simulink model "b07502056_HW5_matlab"  (R2022a)
settings: Solver=VariableStepAuto  StartTime=0.0  StopTime=8  RelTol=1e-3
model workspace (MAT data in the model file):
  Engine_Breakpoint = Simulink.Parameter
  Engine_Breakpoint.Value = [1000 1500 2000 2500 3000 3500 4000 4500 5000 5500 6000 6500 7000 7500 8000 8500 9000]
  Engine_Breakpoint.DataType = 'auto'
  Engine_Breakpoint.Complexity = 'real'
  Engine_Breakpoint.Dimensions = [1 17]
  Engine_Torque = Simulink.Parameter
  Engine_Torque.Value = [850 850 850 850 850 850 850 830 820 770 700 650 600 560 525 490 470]
  Engine_Torque.DataType = 'auto'
  Engine_Torque.Complexity = 'real'
  Engine_Torque.Dimensions = [1 17]
  Final_Drive = 2.5
  Gear_Number = Simulink.Parameter
  Gear_Number.Value = [0 1 2]
  Gear_Number.DataType = 'auto'
  Gear_Number.Complexity = 'real'
  Gear_Number.Dimensions = [1 3]
  Gear_Ratio = Simulink.Parameter
  Gear_Ratio.Value = [-3.297 15.5 8.05]
  Gear_Ratio.DataType = 'auto'
  Gear_Ratio.Complexity = 'real'
  Gear_Ratio.Dimensions = [1 3]
  Pedal_Depth = 1
  Tyre = Simulink.Parameter
  Tyre.Value = [275 0.4 482.6]
  Tyre.DataType = 'auto'
  Tyre.Complexity = 'real'
  Tyre.Dimensions = [1 3]
libraries: vehdynlibviscommon x1, autolibshared x1
settings Model: PacingRate=0.800000  Creator=will  LastModifiedBy=will

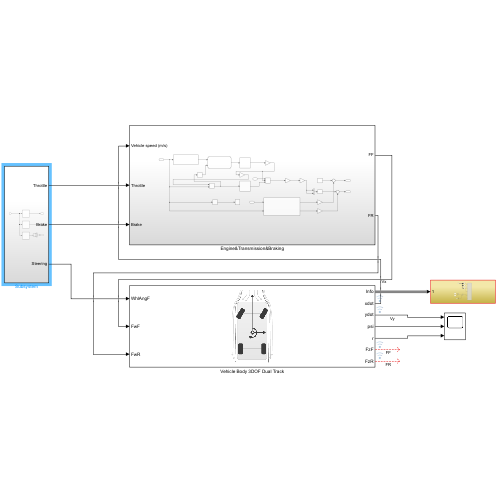
[thumbnail: Simulink's stored preview of the top-level diagram]
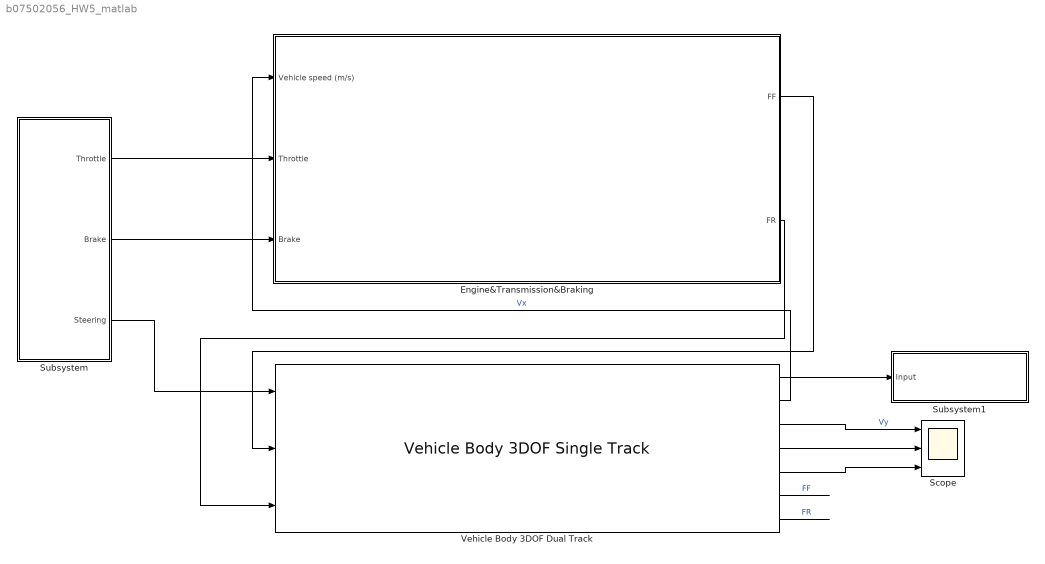
== system b07502056_HW5_matlab ==
  Engine&Transmission&Braking : Subsystem
  Scope : Scope  NumInputPorts=3
  Subsystem : Subsystem
  Subsystem1 : Subsystem
  Vehicle Body 3DOF Dual Track : autolibshared/Vehicle Body 3DOF Single Track  trackMode=Dual  inputMode=External longitudinal forces  frontSteerMode=on  rearSteerMode=off  windMode=off  muMode=off  extFMode=off  extMMode=off  htchFMode=off  htchMMode=off  extXo=off  extpsio=off  extxdoto=off  extro=off  extYo=off  extTamb=off  extydoto=off  aMode=2  NF=2  NR=2  m=2295  a=1.45  b=1.45  h=0.3  dh=1  hh=0.2  X_o=0  xdot_o=0  CalphaMode=off  sigmaMode=on  d=0  hl=0  w=[1.4,1.4]  Cy_f=12e3  Cy_r=11e3  sigma_f=.1  sigma_r=.1  alpha_f_brk=[-.1 .1]  Cy_f_data=[-9e3 9e3]  alpha_r_brk=[-.1 .1]  Cy_r_data=[-9e3 9e3]  Y_o=0  ydot_o=0  Izz=4000  psi_o=0  r_o=0  Af=2.33  Cd=.22  Cl=.1  Cpm=.1  beta_w=[0 0.01:0.01:0.3]  Cs=[0:0.03:0.9]  Cym=[0 1e-6:0.01:0.3]  Pabs=101325  Tair=273  g=9.81  mu=1  xdot_tol=.01  Fznom=5000  Fxtire_sat=7e4  Fytire_sat=7e4  longOff=0  latOff=0  vertOff=0  wrapAng=off
      settings: SourceProductBaseCode=PW,DR,MT,VE
  wires:
  Vehicle Body 3DOF Dual Track/2 -> Engine&Transmission&Braking/1(Vehicle speed (m/s))  "Vx"
  Subsystem/1(Throttle) -> Engine&Transmission&Braking/2(Throttle)
  Engine&Transmission&Braking/2(FR) -> Vehicle Body 3DOF Dual Track/3
  Engine&Transmission&Braking/1(FF) -> Vehicle Body 3DOF Dual Track/2
  Subsystem/2(Brake) -> Engine&Transmission&Braking/3(Brake)
  Subsystem/3(Steering) -> Vehicle Body 3DOF Dual Track/1
  Vehicle Body 3DOF Dual Track/3 -> Scope/1  "Vy"
  Vehicle Body 3DOF Dual Track/4 -> Scope/2
  Vehicle Body 3DOF Dual Track/5 -> Scope/3
  Vehicle Body 3DOF Dual Track/1 -> Subsystem1/1(Input)
  Vehicle Body 3DOF Dual Track/6 -> ?  "FF"
  Vehicle Body 3DOF Dual Track/7 -> ?  "FR"

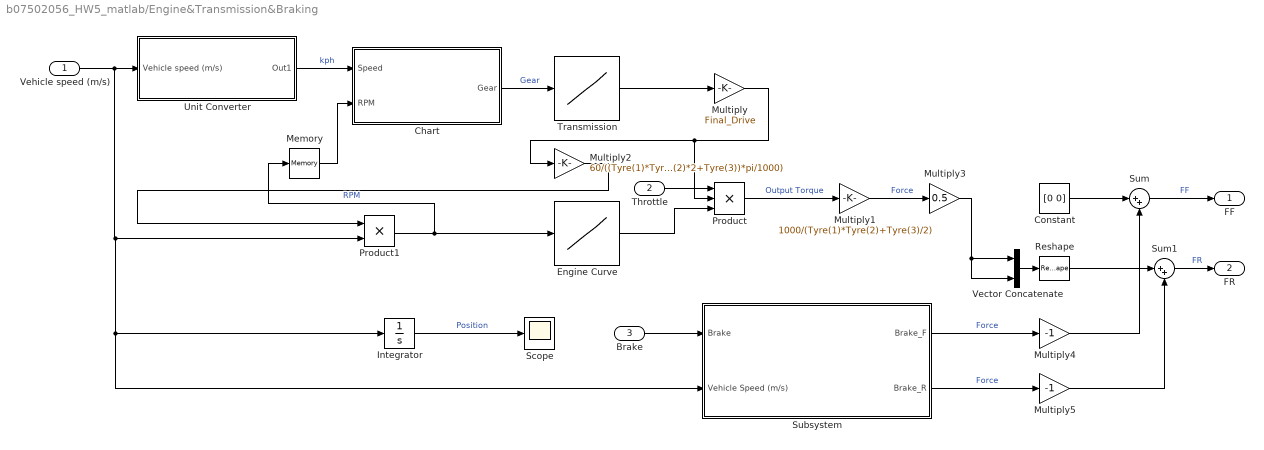
== system b07502056_HW5_matlab/Engine&Transmission&Braking ==
  Vehicle speed (m/s) : Inport
  Throttle : Inport  Port=2
  Brake : Inport  Port=3
  Chart : Stateflow chart  TreatAsAtomicUnit=on
  Constant : Constant  Value=[0 0]
  Engine Curve : Lookup_n-D  NumberOfTableDimensions=1  BreakpointsForDimension1=Engine_Breakpoint  Table=Engine_Torque  InternalRulePriority=Speed  RndMeth=Simplest
  Integrator : Integrator
  Memory : Memory
  Multiply : Gain  Gain=Final_Drive
  Multiply1 : Gain  Gain=1000/(Tyre(1)*Tyre(2)+Tyre(3)/2)
  Multiply2 : Gain  Gain=60/((Tyre(1)*Tyre(2)*2+Tyre(3))*pi/1000)
  Multiply3 : Gain  Gain=0.5
  Multiply4 : Gain  Gain=-1
  Multiply5 : Gain  Gain=-1
  Product : Product  Inputs=3
  Product1 : Product
  Reshape : Reshape
  Scope : Scope
  Subsystem : Subsystem
  Sum : Sum  Inputs=|++
  Sum1 : Sum  Inputs=|++
  Transmission : Lookup_n-D  NumberOfTableDimensions=1  BreakpointsForDimension1=Gear_Number  Table=Gear_Ratio  InternalRulePriority=Speed  RndMeth=Simplest
  Unit Converter : Subsystem
  Vector Concatenate : Concatenate
  FF : Outport
  FR : Outport  Port=2
  wires:
  Chart/1(Gear) -> Transmission/1  "Gear"
  Vehicle speed (m/s)/1 -> Subsystem/2(Vehicle Speed (m/s)), Integrator/1, Product1/2, Unit Converter/1(Vehicle speed (m/s))
  Unit Converter/1(Out1) -> Chart/1(Speed)  "kph"
  Engine Curve/1 -> Product/3
  Transmission/1 -> Multiply/1
  Throttle/1 -> Product/1
  Product/1 -> Multiply1/1  "Output Torque"
  Multiply/1 -> Product/2, Multiply2/1
  Multiply2/1 -> Product1/1
  Product1/1 -> Memory/1, Engine Curve/1  "RPM"
  Memory/1 -> Chart/2(RPM)
  Integrator/1 -> Scope/1  "Position"
  Multiply1/1 -> Multiply3/1  "Force"
  Vector Concatenate/1 -> Reshape/1
  Multiply3/1 -> Vector Concatenate/1, Vector Concatenate/2
  Brake/1 -> Subsystem/1(Brake)
  Sum1/1 -> FR/1  "FR"
  Reshape/1 -> Sum1/1
  Sum/1 -> FF/1  "FF"
  Constant/1 -> Sum/1
  Multiply4/1 -> Sum/2
  Multiply5/1 -> Sum1/2
  Subsystem/1(Brake_F) -> Multiply4/1  "Force"
  Subsystem/2(Brake_R) -> Multiply5/1  "Force"

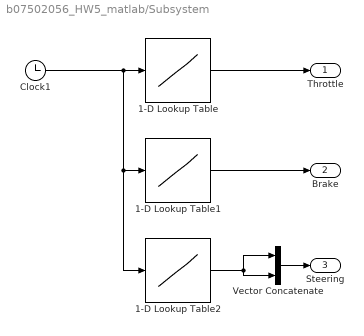
== system b07502056_HW5_matlab/Subsystem ==
  1-D Lookup Table : Lookup_n-D  NumberOfTableDimensions=1  BreakpointsForDimension1=[0;0.49;0.5;2.5;2.6;4;10;15;20]  Table=[0;0;1;1;0;0;1;1;1]  InternalRulePriority=Speed  RndMeth=Simplest
  1-D Lookup Table1 : Lookup_n-D  NumberOfTableDimensions=1  BreakpointsForDimension1=[0;2.5;2.6;2.9;3;20]  Table=[0;0;1;1;0;0]  InternalRulePriority=Speed  RndMeth=Simplest
  1-D Lookup Table2 : Lookup_n-D  NumberOfTableDimensions=1  BreakpointsForDimension1=[0 2.8 2.9 8.3 8.4 20]  Table=[0 0 0.28 0.28 0 0]  InternalRulePriority=Speed  RndMeth=Simplest
  Clock1 : Clock
  Vector Concatenate : Concatenate
  Throttle : Outport
  Brake : Outport  Port=2
  Steering : Outport  Port=3
  wires:
  1-D Lookup Table/1 -> Throttle/1
  1-D Lookup Table1/1 -> Brake/1
  Clock1/1 -> 1-D Lookup Table2/1, 1-D Lookup Table1/1, 1-D Lookup Table/1
  Vector Concatenate/1 -> Steering/1
  1-D Lookup Table2/1 -> Vector Concatenate/1, Vector Concatenate/2

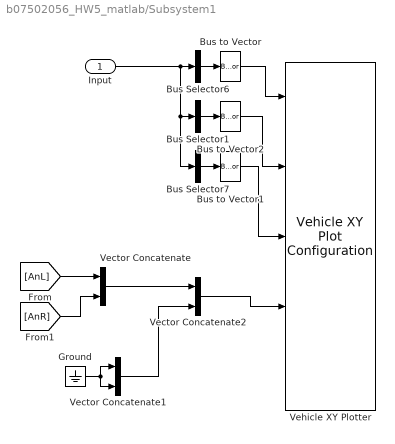
== system b07502056_HW5_matlab/Subsystem1 ==
  Input : Inport
  Bus Selector1 : BusSelector  OutputSignals=InertFrm.Cg.Ang.phi,InertFrm.Cg.Ang.theta,InertFrm.Cg.Ang.psi  OutputAsBus=on
  Bus Selector6 : BusSelector  OutputSignals=InertFrm.Geom.Disp.X,InertFrm.Geom.Disp.Y,InertFrm.Geom.Disp.Z  OutputAsBus=on
  Bus Selector7 : BusSelector  OutputSignals=BdyFrm.Geom.Vel.xdot,BdyFrm.Geom.Vel.ydot,BdyFrm.Geom.Vel.zdot  OutputAsBus=on
  Bus to Vector : BusToVector
  Bus to Vector1 : BusToVector
  Bus to Vector2 : BusToVector
  Ground : Ground
  Vector Concatenate : Concatenate
  Vector Concatenate1 : Concatenate
  Vector Concatenate2 : Concatenate
  Vehicle XY Plotter : vehdynlibviscommon/Vehicle XY Plot Configuration  extRef=on  extStats=off  extTireF=off  a=1.3  b=1.557  w=1.611  figBorder=10  bufferSize=1024  velNorm=5  tireFNorm=1000  pltDT=.1
      settings: SourceProductBaseCode=VE
  wires:
  Input/1 -> Bus Selector7/1, Bus Selector1/1, Bus Selector6/1
  Bus Selector6/1 -> Bus to Vector/1
  Bus to Vector2/1 -> Vehicle XY Plotter/2
  Bus to Vector/1 -> Vehicle XY Plotter/1
  Bus Selector1/1 -> Bus to Vector2/1
  Bus to Vector1/1 -> Vehicle XY Plotter/3
  Bus Selector7/1 -> Bus to Vector1/1
  [AnL] -> Vector Concatenate/1
  [AnR] -> Vector Concatenate/2
  Vector Concatenate/1 -> Vector Concatenate2/1
  Vector Concatenate1/1 -> Vector Concatenate2/2
  Ground/1 -> Vector Concatenate1/1, Vector Concatenate1/2
  Vector Concatenate2/1 -> Vehicle XY Plotter/4

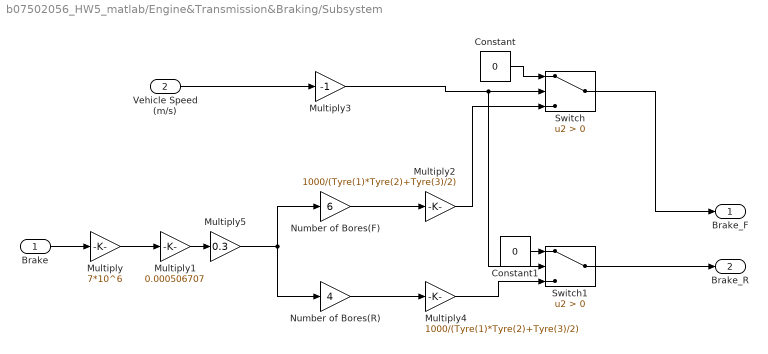
== system b07502056_HW5_matlab/Engine&Transmission&Braking/Subsystem ==
  Brake : Inport
  Vehicle Speed (m/s) : Inport  Port=2
  Constant : Constant  Value=0
  Constant1 : Constant  Value=0
  Multiply : Gain  Gain=7*10^6
  Multiply1 : Gain  Gain=0.000506707
  Multiply2 : Gain  Gain=1000/(Tyre(1)*Tyre(2)+Tyre(3)/2)
  Multiply3 : Gain  Gain=-1
  Multiply4 : Gain  Gain=1000/(Tyre(1)*Tyre(2)+Tyre(3)/2)
  Multiply5 : Gain  Gain=0.3
  Number of Bores(F) : Gain  Gain=6
  Number of Bores(R) : Gain  Gain=4
  Switch : Switch  Criteria=u2 > Threshold  SaturateOnIntegerOverflow=off  InputSameDT=off
  Switch1 : Switch  Criteria=u2 > Threshold  SaturateOnIntegerOverflow=off  InputSameDT=off
  Brake_F : Outport
  Brake_R : Outport  Port=2
  wires:
  Brake/1 -> Multiply/1
  Multiply/1 -> Multiply1/1
  Constant/1 -> Switch/1
  Vehicle Speed (m/s)/1 -> Multiply3/1
  Multiply3/1 -> Switch1/2, Switch/2
  Constant1/1 -> Switch1/1
  Multiply2/1 -> Switch/3
  Multiply4/1 -> Switch1/3
  Switch/1 -> Brake_F/1
  Switch1/1 -> Brake_R/1
  Number of Bores(F)/1 -> Multiply2/1
  Number of Bores(R)/1 -> Multiply4/1
  Multiply1/1 -> Multiply5/1
  Multiply5/1 -> Number of Bores(F)/1, Number of Bores(R)/1

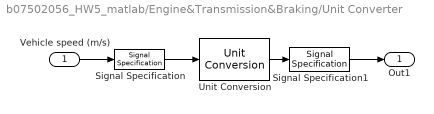
== system b07502056_HW5_matlab/Engine&Transmission&Braking/Unit Converter ==
  Vehicle speed (m/s) : Inport
  Signal Specification : SignalSpecification  Unit=m/s
  Signal Specification1 : SignalSpecification  Unit=km/hr
  Unit Conversion : UnitConversion
  Out1 : Outport
  wires:
  Vehicle speed (m/s)/1 -> Signal Specification/1
  Unit Conversion/1 -> Signal Specification1/1
  Signal Specification/1 -> Unit Conversion/1
  Signal Specification1/1 -> Out1/1

== stateflow chart b07502056_HW5_matlab/Engine&Transmission&Braking/Chart ==
  state Gear1
    Gear=1;
  state Gear2
    Gear=2;
  state Gear3
    Gear=3;
  state Gear4
    Gear=4;
  state Gear5
    Gear=5;
  state Gear8
    Gear=8;
  state Gear7
    Gear=7;
  state Gear6
    Gear=6;
  (default) -> Gear1
  Gear2 -> Gear1 : [RPM<2000]
  Gear4 -> Gear3 [order 2] : [RPM<1000]
  Gear5 -> Gear4 [order 2] : [RPM<1000]
  Gear1 -> Gear2 : [Speed>160||RPM>7000]
  Gear3 -> Gear4 : [Speed>80||RPM>3500]
  Gear4 -> Gear5 [order 1] : [Speed>100||RPM>3500]
  Gear5 -> Gear6 [order 1] : [Speed>120||RPM>3500]
  Gear6 -> Gear5 [order 2] : [RPM<1000]
  Gear7 -> Gear8 [order 1] : [Speed>160||RPM>3500]
  Gear6 -> Gear7 [order 1] : [Speed>140||RPM>3500]
  Gear7 -> Gear6 [order 2] : [RPM<1000]
  Gear8 -> Gear7 : [RPM<1000]
  data: Speed input; RPM input; Gear output
